simulink model "determine_max_speed"  (R2020b)
settings: Solver=ode1  StartTime=0.0  StopTime=20  FixedStep=0.01  RelTol=1e-3  EnableMultiTasking=on
libraries: arduinolib x4
settings Model: SILPILModeSetting=veronly  ExtModeTrigDuration=2  Creator=ONLY-GOD  LastModifiedBy=ONLY-GOD
settings OptimizationCC: EnhancedBackFolding=on  PassReuseOutputArgsAs=Individual arguments  ZeroExternalMemoryAtStartup=off  ZeroInternalMemoryAtStartup=off  MaxStackSize=64  OptimizeBlockOrder=speed  DifferentSizesBufferReuse=on  OptimizationCustomize=off  EfficientTunableParamExpr=on
settings DebuggingCC: ParameterTunabilityLossMsg=error
settings HardwareCC: ProdBitPerPointer=32  ProdBitPerSizeT=32  ProdBitPerPtrDiffT=32  ProdLargestAtomicInteger=Long  ProdLargestAtomicFloat=Double  ProdWordSize=32  ProdHWDeviceType=ARM Compatible->ARM Cortex
settings SFSimCC: MATLABDynamicMemAlloc=off
settings RTWCC: Description=Embedded Coder  SystemTargetFile=ert.tlc  HardwareBoard=Arduino Due  TemplateMakefile=ert_default_tmf  Toolchain=Arduino ARM  BuildConfiguration=Faster Runs
settings CodeAppCC: ForceParamTrailComments=on  IgnoreCustomStorageClasses=off  OperatorAnnotations=on  SimulinkDataObjDesc=on  SFDataObjDesc=on  InsertBlockDesc=on
settings ERTTargetCC: SupportContinuousTime=on  SupportVariableSizeSignals=on  ExtModeTransport=3  ExtModeStaticAllocSize=24576  ExtModeMexFile=ext_xcp  ExtModeIntrfLevel=Level2 - Open

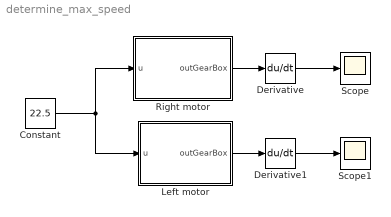
== system determine_max_speed ==
  Constant : Constant  Value=22.5
  Derivative : Derivative
  Derivative1 : Derivative
  Left motor : Subsystem
  Right motor : Subsystem
  Scope : Scope
  Scope1 : Scope
  wires:
  Constant/1 -> Left motor/1(u), Right motor/1(u)
  Right motor/1(outGearBox) -> Derivative/1
  Left motor/1(outGearBox) -> Derivative1/1
  Derivative1/1 -> Scope1/1
  Derivative/1 -> Scope/1

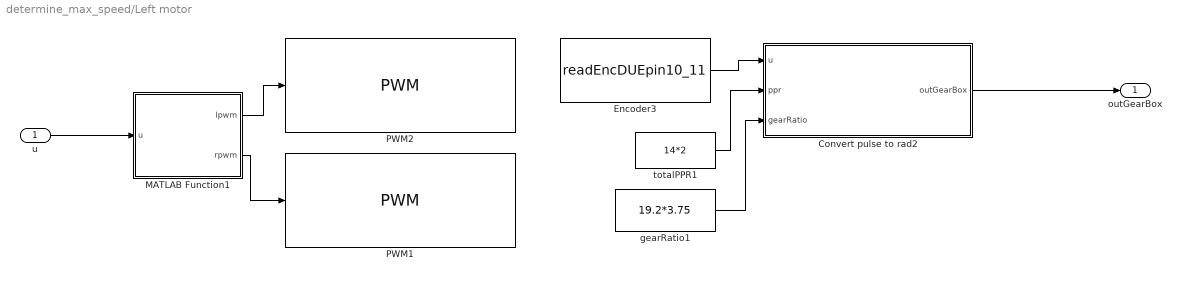
== system determine_max_speed/Left motor ==
  u : Inport
  Convert pulse to rad2 : MATLAB Function  TreatAsAtomicUnit=on
  Encoder3 : S-Function  InitFcn=try, set_param(gcb,'FunctionName','readEncDUEpin10_11'), end  FunctionName=readEncDUEpin10_11  SFunctionModules=readEncDUEpin10_11_wrapper  SFunctionDeploymentMode=off  EnableBusSupport=off  mask(S-Function Builder){}
      mask help: Simulink:masks:SFunctionBuilder_MD
      mask init:
      | val = [[.9  0.75 0.75 1 1 .9 .9 1]',[1 1 0.75 0.75 .9 .9 1 .9]'];try , sys = get_param(gcb,'SfunBuilderFcnName');if isempty(sys), sys = get_param(gcb,'FunctionName'); end,catch, sys = get_param(gcb,'FunctionName'); end
      settings: CopyFcn=set_param(gcbh,'LinkStatus','none')  PreSaveFcn=try, set_param(gcb,'FunctionName','readEncDUEpin10_11'), end  OpenFcn=sfunctionwizard(gcbh)
      mask Display: plot(val(:,1),val(:,2)),disp(sys),port_label('output',1,'countt')
  MATLAB Function1 : MATLAB Function  TreatAsAtomicUnit=on
  PWM1 : arduinolib/PWM  pinNumber=4  frequencyType=Default  desiredFrequency=490.2  achievableFrequency=490.2
  PWM2 : arduinolib/PWM  pinNumber=5  frequencyType=Default  desiredFrequency=490.2  achievableFrequency=490.2
  gearRatio1 : Constant  Value=19.2*3.75
  totalPPR1 : Constant  Value=14*2
  outGearBox : Outport
  wires:
  Encoder3/1 -> Convert pulse to rad2/1(u)
  totalPPR1/1 -> Convert pulse to rad2/2(ppr)
  gearRatio1/1 -> Convert pulse to rad2/3(gearRatio)
  Convert pulse to rad2/1(outGearBox) -> outGearBox/1
  MATLAB Function1/1(lpwm) -> PWM2/1
  MATLAB Function1/2(rpwm) -> PWM1/1
  u/1 -> MATLAB Function1/1(u)

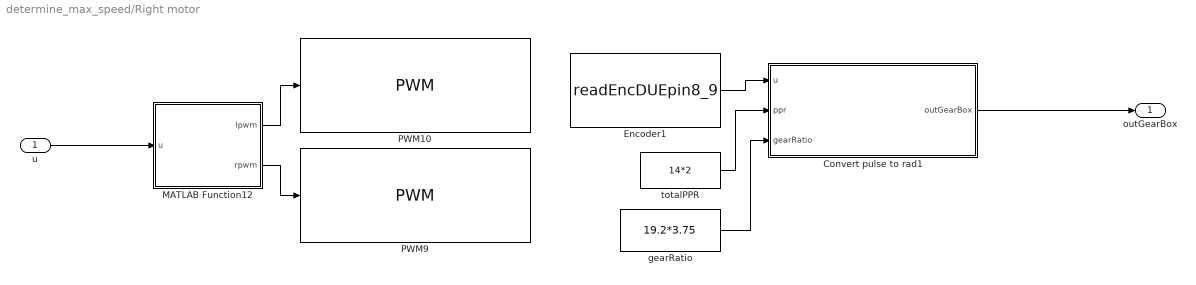
== system determine_max_speed/Right motor ==
  u : Inport
  Convert pulse to rad1 : MATLAB Function  TreatAsAtomicUnit=on
  Encoder1 : S-Function  InitFcn=try, set_param(gcb,'FunctionName','readEncDUEpin8_9'), end  FunctionName=readEncDUEpin8_9  SFunctionModules=readEncDUEpin8_9_wrapper  SFunctionDeploymentMode=off  EnableBusSupport=off  mask(S-Function Builder){}
      mask help: Simulink:masks:SFunctionBuilder_MD
      mask init: same as determine_max_speed/Left motor/Encoder3
      settings: CopyFcn=set_param(gcbh,'LinkStatus','none')  PreSaveFcn=try, set_param(gcb,'FunctionName','readEncDUEpin8_9'), end  OpenFcn=sfunctionwizard(gcbh)
      mask Display: plot(val(:,1),val(:,2)),disp(sys),port_label('output',1,'count')
  MATLAB Function12 : MATLAB Function  TreatAsAtomicUnit=on
  PWM10 : arduinolib/PWM  pinNumber=7  frequencyType=Default  desiredFrequency=490.2  achievableFrequency=490.2
  PWM9 : arduinolib/PWM  pinNumber=6  frequencyType=Default  desiredFrequency=490.2  achievableFrequency=490.2
  gearRatio : Constant  Value=19.2*3.75
  totalPPR : Constant  Value=14*2
  outGearBox : Outport
  wires:
  gearRatio/1 -> Convert pulse to rad1/3(gearRatio)
  MATLAB Function12/2(rpwm) -> PWM9/1
  MATLAB Function12/1(lpwm) -> PWM10/1
  totalPPR/1 -> Convert pulse to rad1/2(ppr)
  Encoder1/1 -> Convert pulse to rad1/1(u)
  Convert pulse to rad1/1(outGearBox) -> outGearBox/1
  u/1 -> MATLAB Function12/1(u)

== matlab function determine_max_speed/Right motor/Convert pulse to rad1 ==
  settings: updateMethod=DISCRETE
  data: u input; ppr input; gearRatio input; outGearBox output
function outGearBox = fcn(u,ppr,gearRatio)

persistent counter_num over_flag
if(isempty(counter_num)), counter_num = 0;end
if(isempty(over_flag)), over_flag = 0;end
pulse2radian = 2*pi/ppr; % 1 pulse = ?? radian

if(double(u) - counter_num > 40000), over_flag = over_flag-1;
elseif(double(u) - counter_num < -40000), over_flag = over_flag+1;
end

inGearBox = (double(u)+over_flag*(2^32 -1))*pulse2radian; 
outGearBox = inGearBox/gearRatio;
counter_num = double(u) ;

== matlab function determine_max_speed/Left motor/Convert pulse to rad2 ==
  settings: updateMethod=DISCRETE
  data: u input; ppr input; gearRatio input; outGearBox output
function outGearBox = fcn(u,ppr,gearRatio)

persistent counter_num over_flag
if(isempty(counter_num)), counter_num = 0;end
if(isempty(over_flag)), over_flag = 0;end
pulse2radian = 2*pi/ppr; % 1 pulse = ?? radian

if(double(u) - counter_num > 40000), over_flag = over_flag-1;
elseif(double(u) - counter_num < -40000), over_flag = over_flag+1;
end

inGearBox = (double(u)+over_flag*(2^32 -1))*pulse2radian; 
outGearBox = inGearBox/gearRatio;
counter_num = double(u) ;

== matlab function determine_max_speed/Right motor/MATLAB Function12 ==
  data: u input; lpwm output; rpwm output
function [lpwm,rpwm] = fcn(u)

Vmax = 22.9;
pwm = u*254/Vmax;
if pwm > 0
    lpwm = pwm;
    rpwm = 0;
elseif pwm < 0
    lpwm = 0;
    rpwm = abs(pwm);
else
    lpwm = 0;
    rpwm = 0;
end

== matlab function determine_max_speed/Left motor/MATLAB Function1 ==
  data: u input; lpwm output; rpwm output
function [lpwm,rpwm] = fcn(u)

Vmax = 22.9;
pwm = u*254/Vmax;
if pwm > 0
    lpwm = pwm;
    rpwm = 0;
elseif pwm < 0
    lpwm = 0;
    rpwm = abs(pwm);
else
    lpwm = 0;
    rpwm = 0;
end
